simulink model "four_tanks_baseline_dT_nonminphase"  (Simulink 7.5)
settings: Solver=ode45  StartTime=0.0  StopTime=simtime  MaxStep=.01  RelTol=1e-3
model workspace (MAT data in the model file):
  gamma_1 : Simulink.Parameter (value not decoded)
  gamma_2 : Simulink.Parameter (value not decoded)
  a1 : Simulink.Parameter (value not decoded)
  a2 : Simulink.Parameter (value not decoded)
  a3 : Simulink.Parameter (value not decoded)
  a4 : Simulink.Parameter (value not decoded)
  g : Simulink.Parameter (value not decoded)
  A_1 : Simulink.Parameter (value not decoded)
  A_2 : Simulink.Parameter (value not decoded)
  A_3 : Simulink.Parameter (value not decoded)
  A_4 : Simulink.Parameter (value not decoded)
  x1o : Simulink.Parameter (value not decoded)
  x2o : Simulink.Parameter (value not decoded)
  x3o : Simulink.Parameter (value not decoded)
  x4o : Simulink.Parameter (value not decoded)
  x1_max : Simulink.Parameter (value not decoded)
  x2_max : Simulink.Parameter (value not decoded)
  x3_max : Simulink.Parameter (value not decoded)
  x4_max : Simulink.Parameter (value not decoded)
  u1_max : Simulink.Parameter (value not decoded)
  u2_max : Simulink.Parameter (value not decoded)
  x1f : Simulink.Parameter (value not decoded)
  x2f : Simulink.Parameter (value not decoded)
  Ts : Simulink.Parameter (value not decoded)
  simtime : Simulink.Parameter (value not decoded)
  Sig : Simulink.Signal (value not decoded)
  Sig1 : Simulink.Signal (value not decoded)
  Sig2 : Simulink.Signal (value not decoded)
  ku : Simulink.Parameter (value not decoded)
values from neighbouring files (symbols this model uses):
  simtime = max( x1_x2_dec.time )    [plot_four_tank.m]    (also in plot_four_tank_together.m; plot_two_tank.m = max( x1_x2_orig.time ))
settings Model: Creator=Administrator  LastModifiedBy=jporter
settings DebuggingCC: StrictBusMsg=Warning

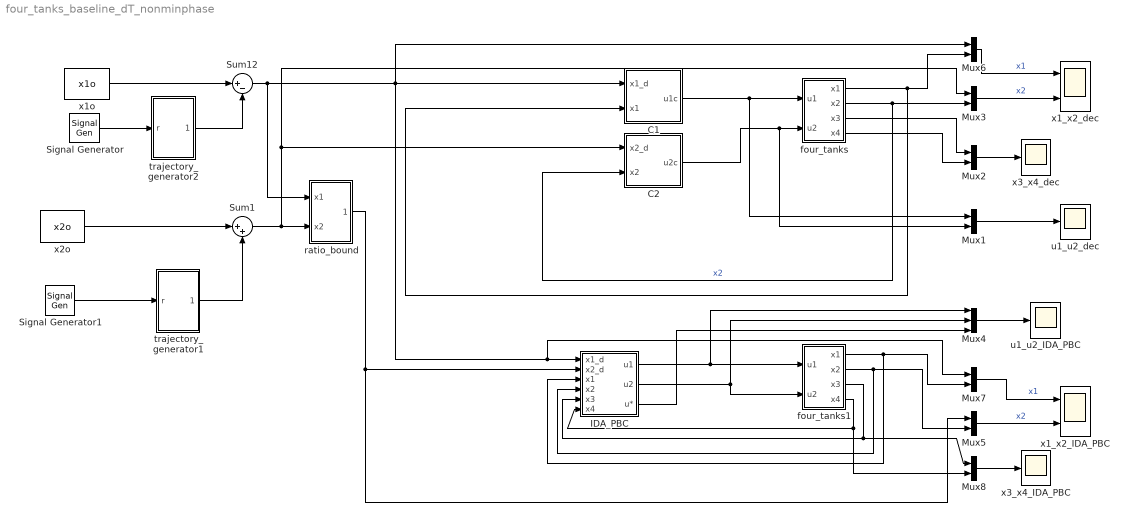
== system four_tanks_baseline_dT_nonminphase ==
  C1 : Subsystem  mask{K=1.5, Ti=110, u1_max=100, gamma_1=gamma_1, gamma_2=gamma_2, x1o=x1o, x2o=x2o, a1=a1, a2=a2, g=g}
      mask prompts: u1_max "u1_max (ml/sec)"
      mask init:
      | L12 = [gamma_1, (1-gamma_2);
      |     (1-gamma_1),gamma_2];
      | us=inv(L12)*[a1*sqrt(2*g*x1o);a2*sqrt(2*g*x2o)];
      | xIo1=us(1)/K
  C2 : Subsystem  mask{K=-0.12, Ti=220, u1_max=100, gamma_1=gamma_1, gamma_2=gamma_2, x1o=x1o, x2o=x2o, a1=a1, a2=a2, g=g}
      mask prompts: u1_max "u2_max (ml/sec)"
      mask init:
      | L12 = [gamma_1, (1-gamma_2);
      |     (1-gamma_1),gamma_2];
      | us=inv(L12)*[a1*sqrt(2*g*x1o);a2*sqrt(2*g*x2o)];
      | xIo2=us(2)/K
  IDA_PBC : Subsystem  mask{k3=5, k4=5, eps1=.75, eps2=.75, epsI1=0.75, epsI2=0.75, A_1=A_1, A_2=A_2, A_3=A_3, A_4=A_4, a1=a1, a2=a2, a3=a3, a4=a4, gamma_1=gamma_1, gamma_2=gamma_2, u1_max=u1_max, u2_max=u2_max, g=g, Ts=Ts, ku=ku}
      mask prompts: eps1 "eps1 (0,1)"; eps2 "eps2 (0,1)"; epsI1 "epsI1 (0,1)"; epsI2 "epsI2 (0,1)"; gamma_1 "gamma_1 in [0,1]"; gamma_2 "gamma_2 in [0,1]"; g "g (cm/s^2)"; Ts "Ts (secs)"
      mask init:
      | if k3 < 0
      |     k3 = 1;
      | end
      | if k4 < 0
      |     k4 = 1;
      | end
      | if (epsI1 <= 0) | (epsI1 >= 1)
      |     epsI1 = .5;
      | end
      | if (epsI2 <= 0) | (epsI2 >= 1)
      |     epsI2 = .5;
      | end
      | kI1 = epsI1*4/A_1;
      | kI2 = epsI2*4/A_2;
      | if (eps1 <= 0) | (eps1 >= 1)
      |     eps1 = .5;
      | end
      | if (eps2 <= 0) | (eps2 >= 1)
      |     eps2 = .5;
      | end
      | k1 = eps1*((4-kI1*A_1)*k3/A_3);
      | k2 = eps2*((4-kI2*A_2)*k4/A_4);
      | JmR=[-1/(k1*A_1),0,1/(k3*A_1),0,0,0;
      |    0,-1/(k2*A_2),0,1/(k4*A_2),0,0;
      |    0,0,-1/(k3*A_3),0,0,0;
      |    0,0,0,-1/(k4*A_4),0,0;
      |    kI1/k1,0,0,0,-kI1/k1,0;
      |    0,kI2/k2,0,0,0,-kI2/k2];
      | eig(JmR+JmR')
      | P=[gamma_1*k1,(1-gamma_1)*k2,0,(1-gamma_1)*k4,gamma_1*k1,(1-gamma_1)*k2;
      |    (1-gamma_2)*k1,gamma_2*k2,(1-gamma_2)*k3,0,(1-gamma_2)*k1,gamma_2*k2];
      | L12=[gamma_1,(1-gamma_2);
      |     (1-gamma_1),gamma_2];
      | L34=[0,(1-gamma_2);
      |     (1-gamma_1),0];
      | Q=eye(2);
      | K=Q*P;
  Mux{1..3,5..8} (7 alike) : Mux  Inputs=2
  Mux4 : Mux  Inputs=[1,1,2]
  Signal Generator : SignalGenerator  WaveForm=square  Amplitude=x1f-x1o  Frequency=2/simtime
  Signal Generator1 : SignalGenerator  WaveForm=square  Amplitude=x2f-x2o+.001  Frequency=2/simtime
  Sum1 : Sum  Inputs=|++  OutDataType=fixdt(1, 16)  OutScaling=2^0
  Sum12 : Sum  Inputs=|+-  OutDataType=fixdt(1, 16)  OutScaling=2^0
  four_tanks : Subsystem  mask{x1o=x1o, x2o=x2o, x3o=x3o, x4o=x4o, x1_max=x1_max, x2_max=x2_max, x3_max=x3_max, x4_max=x4_max, u1_max=u1_max, u2_max=u2_max, a1=a1, a2=a2, a3=a3, a4=a4, A_1=A_1, A_2=A_2, A_3=A_3, A_4=A_4, gamma_1=gamma_1, gamma_2=gamma_2, g=g, ku=ku}
      mask prompts: x1o "x1o (cm)"; x2o "x2o (cm)"; x3o "x3o (cm)"; x4o "x4o (cm)"; x1_max "x1_max (cm)"; x2_max "x2_max (cm)"; x3_max "x3_max (cm)"; x4_max "x4_max (cm)"; u1_max "u1_max (ml/s)"; u2_max "u2_max (ml/s)"; a1 "a1 (cm2)"; a2 "a2 (cm2)"; a3 "a3 (cm2)"; a4 "a4 (cm2)"; A_1 "A_1 (cm2)"; A_2 "A_2 (cm2)"; A_3 "A_3 (cm2)"; A_4 "A_4 (cm2)"; gamma_1 "gamma_1 in [0,1]"; gamma_2 "gamma_2 in [0,1]"; g "g (cm/s2)"
  four_tanks1 : Subsystem  mask{x1o=x1o, x2o=x2o, x3o=x3o, x4o=x4o, x1_max=x1_max, x2_max=x2_max, x3_max=x3_max, x4_max=x4_max, u1_max=u1_max, u2_max=u2_max, a1=a1, a2=a2, a3=a3, a4=a4, A_1=A_1, A_2=A_2, A_3=A_3, A_4=A_4, gamma_1=gamma_1, gamma_2=gamma_2, g=g, ku=ku}
      mask prompts: x1o "x1o (cm)"; x2o "x2o (cm)"; x3o "x3o (cm)"; x4o "x4o (cm)"; x1_max "x1_max (cm)"; x2_max "x2_max (cm)"; x3_max "x3_max (cm)"; x4_max "x4_max (cm)"; u1_max "u1_max (ml/s)"; u2_max "u2_max (ml/s)"; a1 "a1 (cm2)"; a2 "a2 (cm2)"; a3 "a3 (cm2)"; a4 "a4 (cm2)"; A_1 "A_1 (cm2)"; A_2 "A_2 (cm2)"; A_3 "A_3 (cm2)"; A_4 "A_4 (cm2)"; gamma_1 "gamma_1 in [0,1]"; gamma_2 "gamma_2 in [0,1]"; g "g (cm/s2)"
  ratio_bound : Subsystem  mask{gamma_1=gamma_1, gamma_2=gamma_2, a1=a1, a2=a2}
      mask init:
      | x2_x1_max = 0;
      | x2_x1_min = 0;
      | if ( gamma_1 + gamma_2 < 1 )
      |    x2_x1_min = ((a1*gamma_2)/(a2*(1-gamma_2)))^2;
      |    x2_x1_max = ((a1*(1-gamma_1))/(a2*gamma_1))^2;
      | end
      | if ( gamma_1 + gamma_2 > 1 )
      |    x2_x1_min = ((a1*(1-gamma_1))/(a2*gamma_1))^2;
      |    x2_x1_max = ((a1*gamma_2)/(a2 * (1-gamma_2)))^2;
      | end
  trajectory_generator1 : Subsystem  mask{zeta=.9, wn=.05, Ts=Ts}
      mask prompts: zeta "zeta (0 < zeta <= 1)"; wn "wn (radians/sec)"; Ts "Sample Time [Ts] (seconds)"
      mask init:
      | num=[wn^2];
      | den=[1, 2*zeta*wn, wn^2];
      | Hs=tf(num,den);
      | Hz=c2d(Hs,Ts,'tustin');
  trajectory_generator2 : Subsystem  mask{zeta=.9, wn=.05, Ts=Ts}
      mask prompts: zeta "zeta (0 < zeta <= 1)"; wn "wn (radians/sec)"; Ts "Sample Time [Ts] (seconds)"
      mask init:
      | num=[wn^2];
      | den=[1, 2*zeta*wn, wn^2];
      | Hs=tf(num,den);
      | Hz=c2d(Hs,Ts,'tustin');
  u1_u2_IDA_PBC : Scope
      settings: TimeRange=200  YMin=0  YMax=80  SaveName=u1_u2_ida_pbc  SampleInput=on  SampleTime=2
  u1_u2_dec : Scope
      settings: TimeRange=200  YMin=9.5  YMax=12.25  SaveName=u1_u2_dec  SampleInput=on  SampleTime=2
  x1_x2_IDA_PBC : Scope  NumInputPorts=2
      settings: YMin=2.5~5  YMax=17.5~17.5  SaveName=x1_x2_ida_pbc  SampleInput=on  SampleTime=2
  x1_x2_dec : Scope  NumInputPorts=2
      settings: YMin=7.5~0  YMax=22.5~25  SaveName=x1_x2_dec  SampleInput=on  SampleTime=2
  x1o : Constant  Value=x1o  OutDataType=fixdt(1, 16)  OutScaling=2^0  SampleTime=Ts
  x2o : Constant  Value=x2o  OutDataType=fixdt(1, 16)  OutScaling=2^0  SampleTime=Ts
  x3_x4_IDA_PBC : Scope
      settings: TimeRange=200  YMin=0  YMax=17.5  SaveName=x3_x4_ida_pbc  SampleInput=on  SampleTime=2
  x3_x4_dec : Scope
      settings: TimeRange=200  YMin=3.5  YMax=8.5  SaveName=x3_x4_dec  SampleInput=on  SampleTime=2
  wires:
  Signal Generator/1 -> trajectory_generator2/1(r)
  x1o/1 -> Sum12/1
  four_tanks/3(x3) -> Mux2/1
  four_tanks/4(x4) -> Mux2/2
  Mux1/1 -> u1_u2_dec/1
  Mux2/1 -> x3_x4_dec/1
  Sum12/1 -> IDA_PBC/1(x1_d), Mux7/1, Mux6/1, C1/1(x1_d), ratio_bound/1(x1)
  four_tanks/1(x1) -> C1/2(x1), Mux6/2
  four_tanks/2(x2) -> Mux3/2, C2/2(x2)  "x2"
  trajectory_generator2/1(r_traj) -> Sum12/2
  Mux3/1 -> x1_x2_dec/2  "x2"
  Mux6/1 -> x1_x2_dec/1  "x1"
  IDA_PBC/1(u1) -> Mux4/1, four_tanks1/1(u1)
  IDA_PBC/2(u2) -> Mux4/2, four_tanks1/2(u2)
  four_tanks1/4(x4) -> IDA_PBC/6(x4), Mux8/2
  four_tanks1/3(x3) -> IDA_PBC/5(x3), Mux8/1
  four_tanks1/2(x2) -> IDA_PBC/4(x2), Mux5/2
  four_tanks1/1(x1) -> IDA_PBC/3(x1), Mux7/2
  Mux4/1 -> u1_u2_IDA_PBC/1
  IDA_PBC/3(u*) -> Mux4/3
  Mux5/1 -> x1_x2_IDA_PBC/2  "x2"
  Mux7/1 -> x1_x2_IDA_PBC/1  "x1"
  Mux8/1 -> x3_x4_IDA_PBC/1
  x2o/1 -> Sum1/1
  C1/1(u1c) -> Mux1/1, four_tanks/1(u1)
  C2/1(u2c) -> Mux1/2, four_tanks/2(u2)
  Signal Generator1/1 -> trajectory_generator1/1(r)
  trajectory_generator1/1(r_traj) -> Sum1/2
  Sum1/1 -> ratio_bound/2(x2), C2/1(x2_d), Mux3/1
  ratio_bound/1(x2_sat) -> IDA_PBC/2(x2_d), Mux5/1

== system four_tanks_baseline_dT_nonminphase/C1 ==
  x1_d : Inport
  x1 : Inport  Port=2
  1/Ti : Gain  Gain=1/Ti  ParameterDataType=fixdt(1, 16)  ParameterScaling=2^0  OutDataType=fixdt(1, 16)  OutScaling=2^0
  Integrator1 : Integrator  InitialCondition=xIo1  LimitOutput=on  UpperSaturationLimit=u1_max/(abs(K))  LowerSaturationLimit=-u1_max/(abs(K))
  K : Gain  Gain=K  ParameterDataType=fixdt(1, 16)  ParameterScaling=2^0  OutDataType=fixdt(1, 16)  OutScaling=2^0
  SAT : Saturate  UpperLimit=u1_max  LowerLimit=0  OutDataType=fixdt(1, 16)  OutScaling=2^0
  Sum10 : Sum  Inputs=|+-  OutDataType=fixdt(1, 16)  OutScaling=2^0
  Sum11 : Sum  Inputs=++-  OutDataType=fixdt(1, 16)  OutScaling=2^0
  u1c : Outport
  wires:
  K/1 -> SAT/1
  Sum10/1 -> 1/Ti/1
  Sum11/1 -> K/1
  1/Ti/1 -> Integrator1/1
  Integrator1/1 -> Sum11/2
  x1_d/1 -> Sum11/1, Sum10/1
  SAT/1 -> u1c/1
  x1/1 -> Sum10/2, Sum11/3

== system four_tanks_baseline_dT_nonminphase/C2 ==
  x2_d : Inport
  x2 : Inport  Port=2
  1/Ti : Gain  Gain=1/Ti  ParameterDataType=fixdt(1, 16)  ParameterScaling=2^0  OutDataType=fixdt(1, 16)  OutScaling=2^0
  Integrator1 : Integrator  InitialCondition=xIo2  LimitOutput=on  UpperSaturationLimit=u1_max/(abs(K))  LowerSaturationLimit=-u1_max/(abs(K))
  K : Gain  Gain=K  ParameterDataType=fixdt(1, 16)  ParameterScaling=2^0  OutDataType=fixdt(1, 16)  OutScaling=2^0
  SAT : Saturate  UpperLimit=u1_max  LowerLimit=0  OutDataType=fixdt(1, 16)  OutScaling=2^0
  Sum10 : Sum  Inputs=|+-  OutDataType=fixdt(1, 16)  OutScaling=2^0
  Sum11 : Sum  Inputs=++-  OutDataType=fixdt(1, 16)  OutScaling=2^0
  u2c : Outport
  wires:
  x2/1 -> Sum11/3, Sum10/2
  SAT/1 -> u2c/1
  x2_d/1 -> Sum10/1, Sum11/1
  Integrator1/1 -> Sum11/2
  1/Ti/1 -> Integrator1/1
  Sum11/1 -> K/1
  Sum10/1 -> 1/Ti/1
  K/1 -> SAT/1

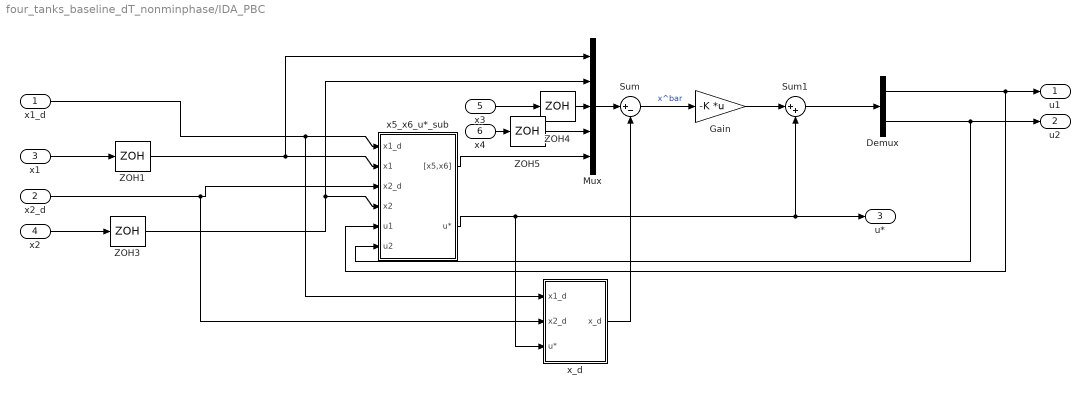
== system four_tanks_baseline_dT_nonminphase/IDA_PBC ==
  x1_d : Inport
  x2_d : Inport  Port=2
  x1 : Inport  Port=3
  x2 : Inport  Port=4
  x3 : Inport  Port=5
  x4 : Inport  Port=6
  Demux : Demux  Outputs=2
  Gain : Gain  Gain=-K  Multiplication=Matrix(K*u)  ParameterDataType=fixdt(1, 16)  ParameterScaling=2^0  OutDataType=fixdt(1, 16)  OutScaling=2^0
  Mux : Mux  Inputs=[1,1,1,1,2]
  Sum : Sum  Inputs=|+-  OutDataType=fixdt(1, 16)  OutScaling=2^0
  Sum1 : Sum  Inputs=|++  OutDataType=fixdt(1, 16)  OutScaling=2^0
  ZOH{1,3..5} (4 alike) : ZeroOrderHold  SampleTime=Ts
  x5_x6_u*_sub : Subsystem
  x_d : Subsystem
  u1 : Outport
  u2 : Outport  Port=2
  u* : Outport  Port=3
  wires:
  x1_d/1 -> x5_x6_u*_sub/1(x1_d), x_d/1(x1_d)
  x1/1 -> ZOH1/1
  x2/1 -> ZOH3/1
  x5_x6_u*_sub/1("[x5,x6]") -> Mux/5
  x3/1 -> ZOH4/1
  x4/1 -> ZOH5/1
  x5_x6_u*_sub/2(u*) -> x_d/3(u*), Sum1/2, u*/1
  Mux/1 -> Sum/1
  x_d/1(x_d) -> Sum/2
  Sum/1 -> Gain/1  "x^bar"
  Gain/1 -> Sum1/1
  Sum1/1 -> Demux/1
  Demux/1 -> u1/1, x5_x6_u*_sub/5(u1)
  Demux/2 -> u2/1, x5_x6_u*_sub/6(u2)
  ZOH1/1 -> Mux/1, x5_x6_u*_sub/2(x1)
  ZOH4/1 -> Mux/3
  ZOH5/1 -> Mux/4
  ZOH3/1 -> x5_x6_u*_sub/4(x2), Mux/2
  x2_d/1 -> x5_x6_u*_sub/3(x2_d), x_d/2(x2_d)

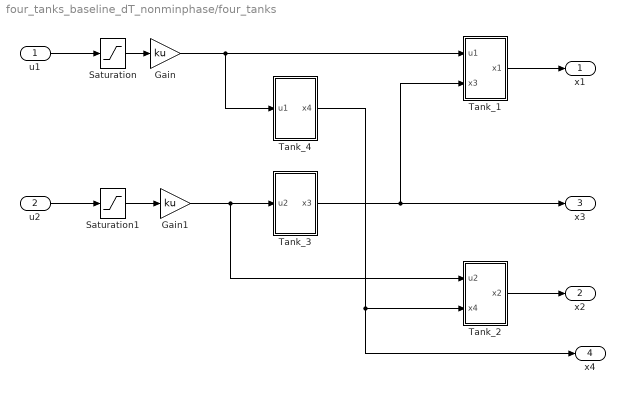
== system four_tanks_baseline_dT_nonminphase/four_tanks ==
  u1 : Inport  OutDataType=fixdt(1, 16)  OutScaling=2^0
  u2 : Inport  Port=2  OutDataType=fixdt(1, 16)  OutScaling=2^0
  Gain : Gain  Gain=ku  ParameterDataType=fixdt(1, 16)  ParameterScaling=2^0  OutDataType=fixdt(1, 16)  OutScaling=2^0
  Gain1 : Gain  Gain=ku  ParameterDataType=fixdt(1, 16)  ParameterScaling=2^0  OutDataType=fixdt(1, 16)  OutScaling=2^0
  Saturation : Saturate  UpperLimit=u1_max  LowerLimit=0  OutDataType=fixdt(1, 16)  OutScaling=2^0
  Saturation1 : Saturate  UpperLimit=u2_max  LowerLimit=0  OutDataType=fixdt(1, 16)  OutScaling=2^0
  Tank_1 : Subsystem
  Tank_2 : Subsystem
  Tank_3 : Subsystem
  Tank_4 : Subsystem
  x1 : Outport  OutDataType=fixdt(1, 16)  OutScaling=2^0
  x2 : Outport  Port=2  OutDataType=fixdt(1, 16)  OutScaling=2^0
  x3 : Outport  Port=3  OutDataType=fixdt(1, 16)  OutScaling=2^0
  x4 : Outport  Port=4  OutDataType=fixdt(1, 16)  OutScaling=2^0
  wires:
  Gain1/1 -> Tank_2/1(u2), Tank_3/1(u2)
  u2/1 -> Saturation1/1
  Gain/1 -> Tank_4/1(u1), Tank_1/1(u1)
  u1/1 -> Saturation/1
  Tank_4/1(x4) -> x4/1, Tank_2/2(x4)
  Tank_3/1(x3) -> x3/1, Tank_1/2(x3)
  Saturation1/1 -> Gain1/1
  Saturation/1 -> Gain/1
  Tank_2/1(x2) -> x2/1
  Tank_1/1(x1) -> x1/1

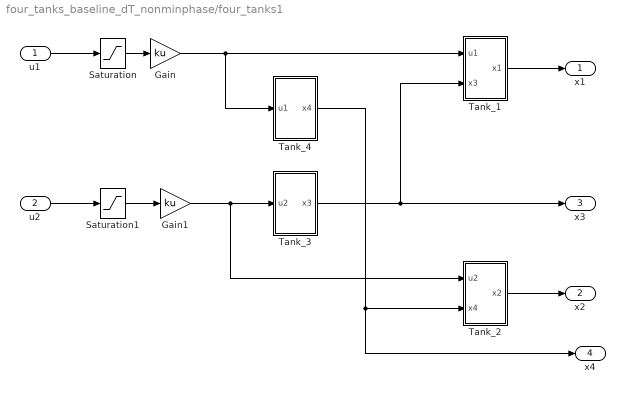
== system four_tanks_baseline_dT_nonminphase/four_tanks1 ==
  u1 : Inport  OutDataType=fixdt(1, 16)  OutScaling=2^0
  u2 : Inport  Port=2  OutDataType=fixdt(1, 16)  OutScaling=2^0
  Gain : Gain  Gain=ku  ParameterDataType=fixdt(1, 16)  ParameterScaling=2^0  OutDataType=fixdt(1, 16)  OutScaling=2^0
  Gain1 : Gain  Gain=ku  ParameterDataType=fixdt(1, 16)  ParameterScaling=2^0  OutDataType=fixdt(1, 16)  OutScaling=2^0
  Saturation : Saturate  UpperLimit=u1_max  LowerLimit=0  OutDataType=fixdt(1, 16)  OutScaling=2^0
  Saturation1 : Saturate  UpperLimit=u2_max  LowerLimit=0  OutDataType=fixdt(1, 16)  OutScaling=2^0
  Tank_1 : Subsystem
  Tank_2 : Subsystem
  Tank_3 : Subsystem
  Tank_4 : Subsystem
  x1 : Outport  OutDataType=fixdt(1, 16)  OutScaling=2^0
  x2 : Outport  Port=2  OutDataType=fixdt(1, 16)  OutScaling=2^0
  x3 : Outport  Port=3  OutDataType=fixdt(1, 16)  OutScaling=2^0
  x4 : Outport  Port=4  OutDataType=fixdt(1, 16)  OutScaling=2^0
  wires:
  Tank_1/1(x1) -> x1/1
  Tank_2/1(x2) -> x2/1
  Saturation/1 -> Gain/1
  Saturation1/1 -> Gain1/1
  Tank_3/1(x3) -> Tank_1/2(x3), x3/1
  Tank_4/1(x4) -> Tank_2/2(x4), x4/1
  u1/1 -> Saturation/1
  Gain/1 -> Tank_1/1(u1), Tank_4/1(u1)
  u2/1 -> Saturation1/1
  Gain1/1 -> Tank_3/1(u2), Tank_2/1(u2)

== system four_tanks_baseline_dT_nonminphase/ratio_bound ==
  x1 : Inport
  x2 : Inport  Port=2
  Divide : Product  Inputs=*/  OutDataType=fixdt(1, 16)  OutScaling=2^-10
  Product : Product  OutDataType=fixdt(1, 16)  OutScaling=2^0  RndMeth=Zero
  Saturation : Saturate  UpperLimit=x2_x1_max  LowerLimit=x2_x1_min  OutDataType=fixdt(1, 16)  OutScaling=2^0
  x2_sat : Outport
  wires:
  Product/1 -> x2_sat/1
  x2/1 -> Divide/1
  x1/1 -> Product/2, Divide/2
  Saturation/1 -> Product/1
  Divide/1 -> Saturation/1

== system four_tanks_baseline_dT_nonminphase/trajectory_generator1 ==
  r : Inport
  Discrete Transfer Fcn : DiscreteTransferFcn  Numerator=Hz.num{1}  Denominator=Hz.den{1}  SampleTime=-1
  ZOH1 : ZeroOrderHold  Priority=-2  SampleTime=Ts
  r_traj : Outport
  wires:
  r/1 -> ZOH1/1
  Discrete Transfer Fcn/1 -> r_traj/1
  ZOH1/1 -> Discrete Transfer Fcn/1

== system four_tanks_baseline_dT_nonminphase/trajectory_generator2 ==
  r : Inport
  Discrete Transfer Fcn : DiscreteTransferFcn  Numerator=Hz.num{1}  Denominator=Hz.den{1}  SampleTime=-1
  ZOH1 : ZeroOrderHold  Priority=-2  SampleTime=Ts
  r_traj : Outport
  wires:
  ZOH1/1 -> Discrete Transfer Fcn/1
  Discrete Transfer Fcn/1 -> r_traj/1
  r/1 -> ZOH1/1

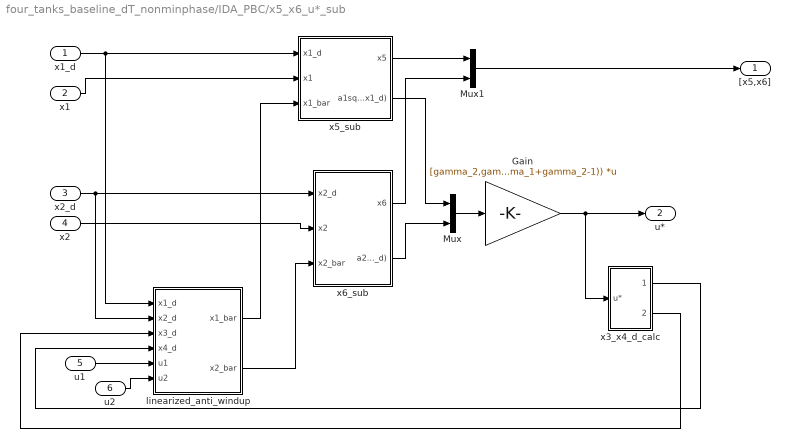
== system four_tanks_baseline_dT_nonminphase/IDA_PBC/x5_x6_u*_sub ==
  x1_d : Inport
  x1 : Inport  Port=2
  x2_d : Inport  Port=3
  x2 : Inport  Port=4
  u1 : Inport  Port=5
  u2 : Inport  Port=6
  Gain : Gain  Gain=[gamma_2,gamma_2-1;gamma_1-1,gamma_1]*(1/(gamma_1+gamma_2-1))  Multiplication=Matrix(K*u)  ParameterDataType=fixdt(1, 16)  ParameterScaling=2^0  OutDataType=fixdt(1, 16)  OutScaling=2^0
  Mux : Mux  Inputs=2
  Mux1 : Mux  Inputs=2
  linearized_anti_windup : Subsystem
  x3_x4_d_calc : Subsystem
  x5_sub : Subsystem
  x6_sub : Subsystem
  "[x5,x6]" : Outport
  u* : Outport  Port=2
  wires:
  x5_sub/2(a1sqrt(2gx1_d)) -> Mux/1
  x6_sub/2(a2sqrt(2gx2_d)) -> Mux/2
  Mux/1 -> Gain/1
  x5_sub/1(x5) -> Mux1/1
  x6_sub/1(x6) -> Mux1/2
  x1_d/1 -> x5_sub/1(x1_d), linearized_anti_windup/1(x1_d)
  Mux1/1 -> "[x5,x6]"/1
  x1/1 -> x5_sub/2(x1)
  x2_d/1 -> x6_sub/1(x2_d), linearized_anti_windup/2(x2_d)
  x2/1 -> x6_sub/2(x2)
  Gain/1 -> u*/1, x3_x4_d_calc/1(u*)
  u2/1 -> linearized_anti_windup/6(u2)
  u1/1 -> linearized_anti_windup/5(u1)
  linearized_anti_windup/2(x2_bar) -> x6_sub/3(x2_bar)
  linearized_anti_windup/1(x1_bar) -> x5_sub/3(x1_bar)
  x3_x4_d_calc/2(x3_d) -> linearized_anti_windup/3(x3_d)
  x3_x4_d_calc/1(x4_d) -> linearized_anti_windup/4(x4_d)

== system four_tanks_baseline_dT_nonminphase/IDA_PBC/x_d ==
  x1_d : Inport
  x2_d : Inport  Port=2
  u* : Inport  Port=3
  Mux1 : Mux  Inputs=[1,1,2,2]
  gen_x3d_x4d : Subsystem
  x5d_x6d : Constant  Value=[0,0]  OutDataType=fixdt(1, 16)  OutScaling=2^0  SampleTime=Ts
  x_d : Outport
  wires:
  x5d_x6d/1 -> Mux1/4
  gen_x3d_x4d/1("[x3d,x4d]") -> Mux1/3
  x1_d/1 -> Mux1/1
  x2_d/1 -> Mux1/2
  Mux1/1 -> x_d/1
  u*/1 -> gen_x3d_x4d/1(u*)

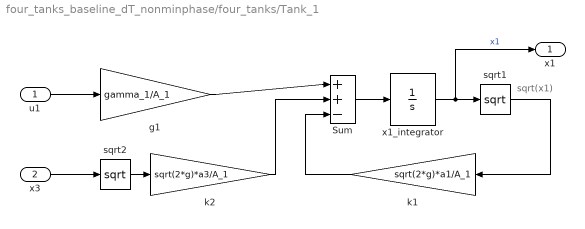
== system four_tanks_baseline_dT_nonminphase/four_tanks/Tank_1 ==
  note: sqrt(x1)
  u1 : Inport
  x3 : Inport  Port=2
  Sum : Sum  Inputs=|++-  OutDataType=fixdt(1, 16)  OutScaling=2^0
  g1 : Gain  Gain=gamma_1/A_1  ParameterDataType=fixdt(1, 16)  ParameterScaling=2^0  OutDataType=fixdt(1, 16)  OutScaling=2^0
  k1 : Gain  Gain=sqrt(2*g)*a1/A_1  ParameterDataType=fixdt(1, 16)  ParameterScaling=2^0  OutDataType=fixdt(1, 16)  OutScaling=2^0
  k2 : Gain  Gain=sqrt(2*g)*a3/A_1  ParameterDataType=fixdt(1, 16)  ParameterScaling=2^0  OutDataType=fixdt(1, 16)  OutScaling=2^0
  sqrt1 : Math  Operator=sqrt  OutDataType=fixdt(1, 16)  OutScaling=2^0  SaturateOnIntegerOverflow=on
  sqrt2 : Math  Operator=sqrt  OutDataType=fixdt(1, 16)  OutScaling=2^0  SaturateOnIntegerOverflow=on
  x1_integrator : Integrator  InitialCondition=x1o  LimitOutput=on  UpperSaturationLimit=x1_max  LowerSaturationLimit=0
  x1 : Outport
  wires:
  k2/1 -> Sum/2
  sqrt2/1 -> k2/1
  x3/1 -> sqrt2/1
  u1/1 -> g1/1
  Sum/1 -> x1_integrator/1
  k1/1 -> Sum/3
  sqrt1/1 -> k1/1
  x1_integrator/1 -> x1/1, sqrt1/1  "x1"
  g1/1 -> Sum/1

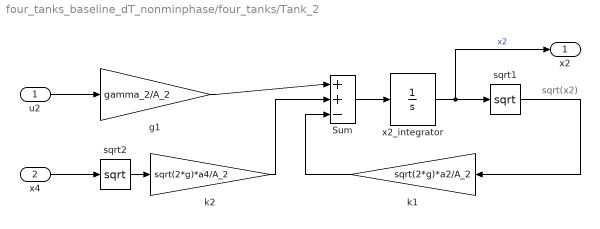
== system four_tanks_baseline_dT_nonminphase/four_tanks/Tank_2 ==
  note: sqrt(x2)
  u2 : Inport
  x4 : Inport  Port=2
  Sum : Sum  Inputs=|++-  OutDataType=fixdt(1, 16)  OutScaling=2^0
  g1 : Gain  Gain=gamma_2/A_2  ParameterDataType=fixdt(1, 16)  ParameterScaling=2^0  OutDataType=fixdt(1, 16)  OutScaling=2^0
  k1 : Gain  Gain=sqrt(2*g)*a2/A_2  ParameterDataType=fixdt(1, 16)  ParameterScaling=2^0  OutDataType=fixdt(1, 16)  OutScaling=2^0
  k2 : Gain  Gain=sqrt(2*g)*a4/A_2  ParameterDataType=fixdt(1, 16)  ParameterScaling=2^0  OutDataType=fixdt(1, 16)  OutScaling=2^0
  sqrt1 : Math  Operator=sqrt  OutDataType=fixdt(1, 16)  OutScaling=2^0  SaturateOnIntegerOverflow=on
  sqrt2 : Math  Operator=sqrt  OutDataType=fixdt(1, 16)  OutScaling=2^0  SaturateOnIntegerOverflow=on
  x2_integrator : Integrator  InitialCondition=x2o  LimitOutput=on  UpperSaturationLimit=x2_max  LowerSaturationLimit=0
  x2 : Outport
  wires:
  g1/1 -> Sum/1
  x2_integrator/1 -> sqrt1/1, x2/1  "x2"
  sqrt1/1 -> k1/1
  k1/1 -> Sum/3
  Sum/1 -> x2_integrator/1
  u2/1 -> g1/1
  x4/1 -> sqrt2/1
  sqrt2/1 -> k2/1
  k2/1 -> Sum/2

== system four_tanks_baseline_dT_nonminphase/four_tanks/Tank_3 ==
  note: sqrt(x3)
  u2 : Inport
  Sum : Sum  Inputs=|+-  OutDataType=fixdt(1, 16)  OutScaling=2^0
  g1 : Gain  Gain=(1-gamma_2)/A_3  ParameterDataType=fixdt(1, 16)  ParameterScaling=2^0  OutDataType=fixdt(1, 16)  OutScaling=2^0
  k1 : Gain  Gain=sqrt(2*g)*a3/A_3  ParameterDataType=fixdt(1, 16)  ParameterScaling=2^0  OutDataType=fixdt(1, 16)  OutScaling=2^0
  sqrt1 : Math  Operator=sqrt  OutDataType=fixdt(1, 16)  OutScaling=2^0  SaturateOnIntegerOverflow=on
  x3_integrator : Integrator  InitialCondition=x3o  LimitOutput=on  UpperSaturationLimit=x3_max  LowerSaturationLimit=0
  x3 : Outport
  wires:
  k1/1 -> Sum/2
  u2/1 -> g1/1
  Sum/1 -> x3_integrator/1
  sqrt1/1 -> k1/1
  x3_integrator/1 -> x3/1, sqrt1/1  "x3"
  g1/1 -> Sum/1

== system four_tanks_baseline_dT_nonminphase/four_tanks/Tank_4 ==
  note: sqrt(x4)
  u1 : Inport
  Sum : Sum  Inputs=|+-  OutDataType=fixdt(1, 16)  OutScaling=2^0
  g1 : Gain  Gain=(1-gamma_1)/A_4  ParameterDataType=fixdt(1, 16)  ParameterScaling=2^0  OutDataType=fixdt(1, 16)  OutScaling=2^0
  k1 : Gain  Gain=sqrt(2*g)*a4/A_4  ParameterDataType=fixdt(1, 16)  ParameterScaling=2^0  OutDataType=fixdt(1, 16)  OutScaling=2^0
  sqrt1 : Math  Operator=sqrt  OutDataType=fixdt(1, 16)  OutScaling=2^0  SaturateOnIntegerOverflow=on
  x4_integrator : Integrator  InitialCondition=x4o  LimitOutput=on  UpperSaturationLimit=x4_max  LowerSaturationLimit=0
  x4 : Outport
  wires:
  g1/1 -> Sum/1
  x4_integrator/1 -> sqrt1/1, x4/1  "x4"
  sqrt1/1 -> k1/1
  Sum/1 -> x4_integrator/1
  u1/1 -> g1/1
  k1/1 -> Sum/2

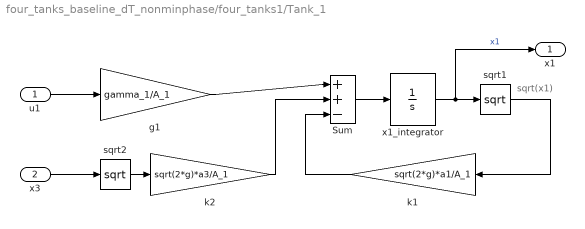
== system four_tanks_baseline_dT_nonminphase/four_tanks1/Tank_1 ==
  note: sqrt(x1)
  u1 : Inport
  x3 : Inport  Port=2
  Sum : Sum  Inputs=|++-  OutDataType=fixdt(1, 16)  OutScaling=2^0
  g1 : Gain  Gain=gamma_1/A_1  ParameterDataType=fixdt(1, 16)  ParameterScaling=2^0  OutDataType=fixdt(1, 16)  OutScaling=2^0
  k1 : Gain  Gain=sqrt(2*g)*a1/A_1  ParameterDataType=fixdt(1, 16)  ParameterScaling=2^0  OutDataType=fixdt(1, 16)  OutScaling=2^0
  k2 : Gain  Gain=sqrt(2*g)*a3/A_1  ParameterDataType=fixdt(1, 16)  ParameterScaling=2^0  OutDataType=fixdt(1, 16)  OutScaling=2^0
  sqrt1 : Math  Operator=sqrt  OutDataType=fixdt(1, 16)  OutScaling=2^0  SaturateOnIntegerOverflow=on
  sqrt2 : Math  Operator=sqrt  OutDataType=fixdt(1, 16)  OutScaling=2^0  SaturateOnIntegerOverflow=on
  x1_integrator : Integrator  InitialCondition=x1o  LimitOutput=on  UpperSaturationLimit=x1_max  LowerSaturationLimit=0
  x1 : Outport
  wires:
  g1/1 -> Sum/1
  x1_integrator/1 -> sqrt1/1, x1/1  "x1"
  sqrt1/1 -> k1/1
  k1/1 -> Sum/3
  Sum/1 -> x1_integrator/1
  u1/1 -> g1/1
  x3/1 -> sqrt2/1
  sqrt2/1 -> k2/1
  k2/1 -> Sum/2

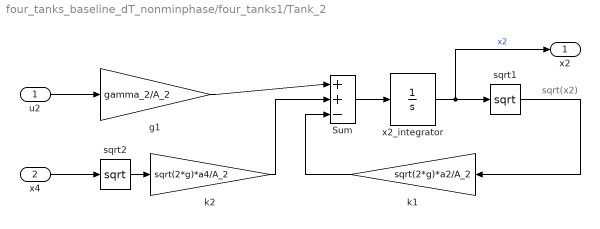
== system four_tanks_baseline_dT_nonminphase/four_tanks1/Tank_2 ==
  note: sqrt(x2)
  u2 : Inport
  x4 : Inport  Port=2
  Sum : Sum  Inputs=|++-  OutDataType=fixdt(1, 16)  OutScaling=2^0
  g1 : Gain  Gain=gamma_2/A_2  ParameterDataType=fixdt(1, 16)  ParameterScaling=2^0  OutDataType=fixdt(1, 16)  OutScaling=2^0
  k1 : Gain  Gain=sqrt(2*g)*a2/A_2  ParameterDataType=fixdt(1, 16)  ParameterScaling=2^0  OutDataType=fixdt(1, 16)  OutScaling=2^0
  k2 : Gain  Gain=sqrt(2*g)*a4/A_2  ParameterDataType=fixdt(1, 16)  ParameterScaling=2^0  OutDataType=fixdt(1, 16)  OutScaling=2^0
  sqrt1 : Math  Operator=sqrt  OutDataType=fixdt(1, 16)  OutScaling=2^0  SaturateOnIntegerOverflow=on
  sqrt2 : Math  Operator=sqrt  OutDataType=fixdt(1, 16)  OutScaling=2^0  SaturateOnIntegerOverflow=on
  x2_integrator : Integrator  InitialCondition=x2o  LimitOutput=on  UpperSaturationLimit=x2_max  LowerSaturationLimit=0
  x2 : Outport
  wires:
  k2/1 -> Sum/2
  sqrt2/1 -> k2/1
  x4/1 -> sqrt2/1
  u2/1 -> g1/1
  Sum/1 -> x2_integrator/1
  k1/1 -> Sum/3
  sqrt1/1 -> k1/1
  x2_integrator/1 -> x2/1, sqrt1/1  "x2"
  g1/1 -> Sum/1

== system four_tanks_baseline_dT_nonminphase/four_tanks1/Tank_3 ==
  note: sqrt(x3)
  u2 : Inport
  Sum : Sum  Inputs=|+-  OutDataType=fixdt(1, 16)  OutScaling=2^0
  g1 : Gain  Gain=(1-gamma_2)/A_3  ParameterDataType=fixdt(1, 16)  ParameterScaling=2^0  OutDataType=fixdt(1, 16)  OutScaling=2^0
  k1 : Gain  Gain=sqrt(2*g)*a3/A_3  ParameterDataType=fixdt(1, 16)  ParameterScaling=2^0  OutDataType=fixdt(1, 16)  OutScaling=2^0
  sqrt1 : Math  Operator=sqrt  OutDataType=fixdt(1, 16)  OutScaling=2^0  SaturateOnIntegerOverflow=on
  x3_integrator : Integrator  InitialCondition=x3o  LimitOutput=on  UpperSaturationLimit=x3_max  LowerSaturationLimit=0
  x3 : Outport
  wires:
  g1/1 -> Sum/1
  x3_integrator/1 -> sqrt1/1, x3/1  "x3"
  sqrt1/1 -> k1/1
  Sum/1 -> x3_integrator/1
  u2/1 -> g1/1
  k1/1 -> Sum/2

== system four_tanks_baseline_dT_nonminphase/four_tanks1/Tank_4 ==
  note: sqrt(x4)
  u1 : Inport
  Sum : Sum  Inputs=|+-  OutDataType=fixdt(1, 16)  OutScaling=2^0
  g1 : Gain  Gain=(1-gamma_1)/A_4  ParameterDataType=fixdt(1, 16)  ParameterScaling=2^0  OutDataType=fixdt(1, 16)  OutScaling=2^0
  k1 : Gain  Gain=sqrt(2*g)*a4/A_4  ParameterDataType=fixdt(1, 16)  ParameterScaling=2^0  OutDataType=fixdt(1, 16)  OutScaling=2^0
  sqrt1 : Math  Operator=sqrt  OutDataType=fixdt(1, 16)  OutScaling=2^0  SaturateOnIntegerOverflow=on
  x4_integrator : Integrator  InitialCondition=x4o  LimitOutput=on  UpperSaturationLimit=x4_max  LowerSaturationLimit=0
  x4 : Outport
  wires:
  k1/1 -> Sum/2
  u1/1 -> g1/1
  Sum/1 -> x4_integrator/1
  sqrt1/1 -> k1/1
  x4_integrator/1 -> x4/1, sqrt1/1  "x4"
  g1/1 -> Sum/1

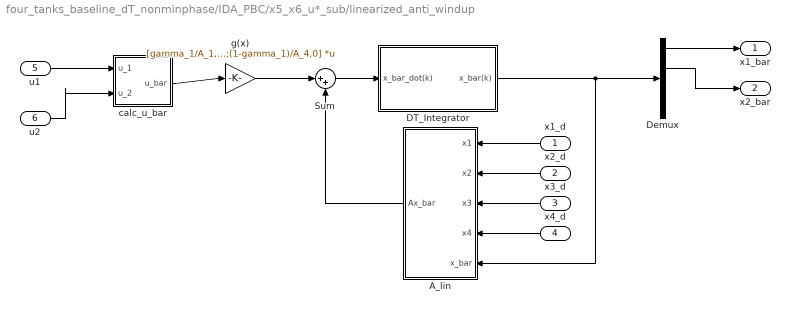
== system four_tanks_baseline_dT_nonminphase/IDA_PBC/x5_x6_u*_sub/linearized_anti_windup ==
  x1_d : Inport
  x2_d : Inport  Port=2
  x3_d : Inport  Port=3
  x4_d : Inport  Port=4
  u1 : Inport  Port=5
  u2 : Inport  Port=6
  A_lin : Stateflow chart  TreatAsAtomicUnit=on
  DT_Integrator : Subsystem
  Demux : Demux
  Sum : Sum  Inputs=|++  OutDataType=fixdt(1, 16)  OutScaling=2^0
  calc_u_bar : Subsystem
  g(x) : Gain  Gain=[gamma_1/A_1,0;0,gamma_2/A_2;0,(1-gamma_2)/A_3;(1-gamma_1)/A_4,0]  Multiplication=Matrix(K*u)  ParameterDataType=fixdt(1, 16)  ParameterScaling=2^0  OutDataType=fixdt(1, 16)  OutScaling=2^0
  x1_bar : Outport
  x2_bar : Outport  Port=2
  wires:
  DT_Integrator/1(x_bar(k)) -> Demux/1, A_lin/5(x_bar)
  Demux/1 -> x1_bar/1
  Demux/2 -> x2_bar/1
  Sum/1 -> DT_Integrator/1(x_bar_dot(k))
  x1_d/1 -> A_lin/1(x1)
  x2_d/1 -> A_lin/2(x2)
  x3_d/1 -> A_lin/3(x3)
  x4_d/1 -> A_lin/4(x4)
  A_lin/1(Ax_bar) -> Sum/2
  calc_u_bar/1(u_bar) -> g(x)/1
  u1/1 -> calc_u_bar/1(u_1)
  u2/1 -> calc_u_bar/2(u_2)
  g(x)/1 -> Sum/1

== system four_tanks_baseline_dT_nonminphase/IDA_PBC/x5_x6_u*_sub/x3_x4_d_calc ==
  u* : Inport
  Demux : Demux  Outputs=2
  Gain1 : Gain  Gain=(1-gamma_2)^2/(2*g*a3^2)  Multiplication=Matrix(K*u)  ParameterDataType=fixdt(1, 16)  ParameterScaling=2^0  OutDataType=fixdt(1, 16)  OutScaling=2^0
  Gain2 : Gain  Gain=(1-gamma_1)^2/(2*g*a4^2)  Multiplication=Matrix(K*u)  ParameterDataType=fixdt(1, 16)  ParameterScaling=2^0  OutDataType=fixdt(1, 16)  OutScaling=2^0
  Product : Product  OutDataType=fixdt(1, 16)  OutScaling=2^0  RndMeth=Zero
  Product1 : Product  OutDataType=fixdt(1, 16)  OutScaling=2^0  RndMeth=Zero
  x4_d : Outport
  x3_d : Outport  Port=2
  wires:
  Demux/1 -> Product/1, Product/2
  Demux/2 -> Product1/1, Product1/2
  Product1/1 -> Gain1/1
  Product/1 -> Gain2/1
  u*/1 -> Demux/1
  Gain2/1 -> x4_d/1
  Gain1/1 -> x3_d/1

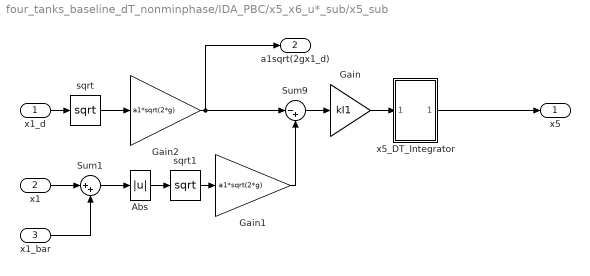
== system four_tanks_baseline_dT_nonminphase/IDA_PBC/x5_x6_u*_sub/x5_sub ==
  x1_d : Inport
  x1 : Inport  Port=2
  x1_bar : Inport  Port=3
  Abs : Abs  OutDataType=fixdt(1, 16)  OutScaling=2^0
  Gain : Gain  Gain=kI1  ParameterDataType=fixdt(1, 16)  ParameterScaling=2^0  OutDataType=fixdt(1, 16)  OutScaling=2^0
  Gain1 : Gain  Gain=a1*sqrt(2*g)  ParameterDataType=fixdt(1, 16)  ParameterScaling=2^0  OutDataType=fixdt(1, 16)  OutScaling=2^0
  Gain2 : Gain  Gain=a1*sqrt(2*g)  ParameterDataType=fixdt(1, 16)  ParameterScaling=2^0  OutDataType=fixdt(1, 16)  OutScaling=2^0
  Sum1 : Sum  Inputs=|++  OutDataType=fixdt(1, 16)  OutScaling=2^0
  Sum9 : Sum  Inputs=|-+  OutDataType=fixdt(1, 16)  OutScaling=2^0
  sqrt : Math  Operator=sqrt  OutDataType=fixdt(1, 16)  OutScaling=2^0  SaturateOnIntegerOverflow=on
  sqrt1 : Math  Operator=sqrt  OutDataType=fixdt(1, 16)  OutScaling=2^0  SaturateOnIntegerOverflow=on
  x5_DT_Integrator : Subsystem
  x5 : Outport
  a1sqrt(2gx1_d) : Outport  Port=2
  wires:
  sqrt/1 -> Gain2/1
  Sum9/1 -> Gain/1
  x1_d/1 -> sqrt/1
  x5_DT_Integrator/1(Out1) -> x5/1
  Gain1/1 -> Sum9/2
  Gain2/1 -> Sum9/1, a1sqrt(2gx1_d)/1
  Gain/1 -> x5_DT_Integrator/1(In1)
  sqrt1/1 -> Gain1/1
  x1/1 -> Sum1/1
  x1_bar/1 -> Sum1/2
  Abs/1 -> sqrt1/1
  Sum1/1 -> Abs/1

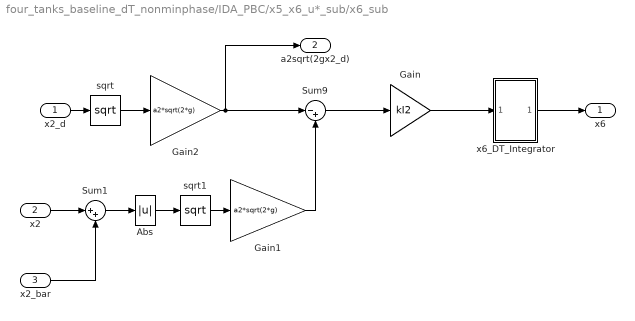
== system four_tanks_baseline_dT_nonminphase/IDA_PBC/x5_x6_u*_sub/x6_sub ==
  x2_d : Inport
  x2 : Inport  Port=2
  x2_bar : Inport  Port=3
  Abs : Abs  OutDataType=fixdt(1, 16)  OutScaling=2^0
  Gain : Gain  Gain=kI2  ParameterDataType=fixdt(1, 16)  ParameterScaling=2^0  OutDataType=fixdt(1, 16)  OutScaling=2^0
  Gain1 : Gain  Gain=a2*sqrt(2*g)  ParameterDataType=fixdt(1, 16)  ParameterScaling=2^0  OutDataType=fixdt(1, 16)  OutScaling=2^0
  Gain2 : Gain  Gain=a2*sqrt(2*g)  ParameterDataType=fixdt(1, 16)  ParameterScaling=2^0  OutDataType=fixdt(1, 16)  OutScaling=2^0
  Sum1 : Sum  Inputs=|++  OutDataType=fixdt(1, 16)  OutScaling=2^0
  Sum9 : Sum  Inputs=|-+  OutDataType=fixdt(1, 16)  OutScaling=2^0
  sqrt : Math  Operator=sqrt  OutDataType=fixdt(1, 16)  OutScaling=2^0  SaturateOnIntegerOverflow=on
  sqrt1 : Math  Operator=sqrt  OutDataType=fixdt(1, 16)  OutScaling=2^0  SaturateOnIntegerOverflow=on
  x6_DT_Integrator : Subsystem
  x6 : Outport
  a2sqrt(2gx2_d) : Outport  Port=2
  wires:
  Gain2/1 -> a2sqrt(2gx2_d)/1, Sum9/1
  Gain1/1 -> Sum9/2
  x6_DT_Integrator/1(Out1) -> x6/1
  x2_d/1 -> sqrt/1
  Sum9/1 -> Gain/1
  sqrt/1 -> Gain2/1
  Gain/1 -> x6_DT_Integrator/1(In1)
  sqrt1/1 -> Gain1/1
  x2/1 -> Sum1/1
  Sum1/1 -> Abs/1
  Abs/1 -> sqrt1/1
  x2_bar/1 -> Sum1/2

== system four_tanks_baseline_dT_nonminphase/IDA_PBC/x_d/gen_x3d_x4d ==
  u* : Inport
  L1 : Gain  Gain=1/(2*g)  ParameterDataType=fixdt(1, 16)  ParameterScaling=2^0  OutDataType=fixdt(1, 16)  OutScaling=2^0
  L34 : Gain  Gain=L34  Multiplication=Matrix(K*u)  ParameterDataType=fixdt(1, 16)  ParameterScaling=2^0  OutDataType=fixdt(1, 16)  OutScaling=2^0
  Product : Product  OutDataType=fixdt(1, 16)  OutScaling=2^0  RndMeth=Zero
  scale : Gain  Gain=[1/a3,0;0,1/a4]  Multiplication=Matrix(K*u)  ParameterDataType=fixdt(1, 16)  ParameterScaling=2^0  OutDataType=fixdt(1, 16)  OutScaling=2^0
  "[x3d,x4d]" : Outport
  wires:
  L34/1 -> scale/1
  scale/1 -> Product/2, Product/1
  Product/1 -> L1/1
  L1/1 -> "[x3d,x4d]"/1
  u*/1 -> L34/1

== system four_tanks_baseline_dT_nonminphase/IDA_PBC/x5_x6_u*_sub/linearized_anti_windup/DT_Integrator ==
  x_bar_dot(k) : Inport
  Sum2 : Sum  Inputs=|++  OutDataType=fixdt(1, 16)  OutScaling=2^0
  Sum3 : Sum  Inputs=|++  OutDataType=fixdt(1, 16)  OutScaling=2^0
  Ts/2 : Gain  Gain=Ts/2  ParameterDataType=fixdt(1, 16)  ParameterScaling=2^0  OutDataType=fixdt(1, 16)  OutScaling=2^0
  Unit Delay1 : UnitDelay  SampleTime=Ts
  Unit Delay3 : UnitDelay  SampleTime=Ts
  x_bar(k) : Outport
  wires:
  Ts/2/1 -> Sum3/1
  Unit Delay1/1 -> x_bar(k)/1, Sum3/2  "xI1(k)"
  Sum3/1 -> Unit Delay1/1  "xI1(k+1)"
  Sum2/1 -> Ts/2/1
  Unit Delay3/1 -> Sum2/1  "xI1_dot(k)"
  x_bar_dot(k)/1 -> Unit Delay3/1, Sum2/2

== system four_tanks_baseline_dT_nonminphase/IDA_PBC/x5_x6_u*_sub/linearized_anti_windup/calc_u_bar ==
  u_1 : Inport
  u_2 : Inport  Port=2
  Mux : Mux  Inputs=2
  Saturation : Saturate  UpperLimit=[u1_max,u2_max]  LowerLimit=[0,0]  OutDataType=fixdt(1, 16)  OutScaling=2^0
  Sum1 : Sum  Inputs=+-  OutDataType=fixdt(1, 16)  OutScaling=2^0
  u_bar : Outport
  wires:
  Saturation/1 -> Sum1/2
  Mux/1 -> Saturation/1, Sum1/1
  u_1/1 -> Mux/1
  u_2/1 -> Mux/2
  Sum1/1 -> u_bar/1

== system four_tanks_baseline_dT_nonminphase/IDA_PBC/x5_x6_u*_sub/x5_sub/x5_DT_Integrator ==
  In1 : Inport
  Sum2 : Sum  Inputs=|++  OutDataType=fixdt(1, 16)  OutScaling=2^0
  Sum3 : Sum  Inputs=|++  OutDataType=fixdt(1, 16)  OutScaling=2^0
  Ts/2 : Gain  Gain=Ts/2  ParameterDataType=fixdt(1, 16)  ParameterScaling=2^0  OutDataType=fixdt(1, 16)  OutScaling=2^0
  Unit Delay1 : UnitDelay  SampleTime=-1
  Unit Delay3 : UnitDelay  SampleTime=-1
  Out1 : Outport
  wires:
  In1/1 -> Sum2/2, Unit Delay3/1
  Unit Delay3/1 -> Sum2/1  "xI1_dot(k)"
  Sum2/1 -> Ts/2/1
  Sum3/1 -> Unit Delay1/1  "xI1(k+1)"
  Unit Delay1/1 -> Sum3/2, Out1/1  "xI1(k)"
  Ts/2/1 -> Sum3/1

== system four_tanks_baseline_dT_nonminphase/IDA_PBC/x5_x6_u*_sub/x6_sub/x6_DT_Integrator ==
  In1 : Inport
  Sum2 : Sum  Inputs=|++  OutDataType=fixdt(1, 16)  OutScaling=2^0
  Sum3 : Sum  Inputs=|++  OutDataType=fixdt(1, 16)  OutScaling=2^0
  Ts/2 : Gain  Gain=Ts/2  ParameterDataType=fixdt(1, 16)  ParameterScaling=2^0  OutDataType=fixdt(1, 16)  OutScaling=2^0
  Unit Delay1 : UnitDelay  SampleTime=-1
  Unit Delay3 : UnitDelay  SampleTime=-1
  Out1 : Outport
  wires:
  In1/1 -> Sum2/2, Unit Delay3/1
  Unit Delay3/1 -> Sum2/1  "xI1_dot(k)"
  Sum2/1 -> Ts/2/1
  Sum3/1 -> Unit Delay1/1  "xI1(k+1)"
  Unit Delay1/1 -> Sum3/2, Out1/1  "xI1(k)"
  Ts/2/1 -> Sum3/1

== matlab function IDA_PBC/x5_x6_u*_sub/linearized_anti_windup/A_lin ==
  settings: updateMethod=DISCRETE  sampleTime=Ts
  data: x1 input double; x2 input double; x3 input double; x4 input double; x_bar input double; Ax_bar output double; g parameter double; a1 parameter double; a2 parameter double; a3 parameter double; a4 parameter double; A_1 parameter double; A_2 parameter double; A_3 parameter double; A_4 parameter double
function Ax_bar  = fcn(x1, x2, x3, x4, x_bar, g, a1, a2, a3, a4, A_1, A_2, A_3, A_4)
x_min = 1;
if x1 < x_min
    x1 = 1;
end
if x2 < x_min
    x2 = x_min;
end
if x3 < x_min
    x3 = x_min;
end
if x4 < x_min
    x4 = x_min;
end
A =[-a1/(A_1*sqrt(x1)), 0, a3/(A_1*sqrt(x3)), 0;
0, -a2/(A_2*sqrt(x2)), 0, a4/(A_2*sqrt(x4));
0, 0, -a3/(A_3*sqrt(x3)), 0;
0, 0, 0, -a4/(A_4*sqrt(x4))];
A = (1/2)*sqrt(2*g)*A;
Ax_bar = A*x_bar;
